simulink model "SymbolSyncTest"  (R2022b)
settings: Solver=VariableStepAuto  StartTime=0.0  StopTime=10.0  RelTol=1e-3
libraries: commfilt2 x2, commrandsrc3 x1, commdigbbndpm3 x1, dspsigops x1
settings Model: Creator=svdvl  LastModifiedBy=User

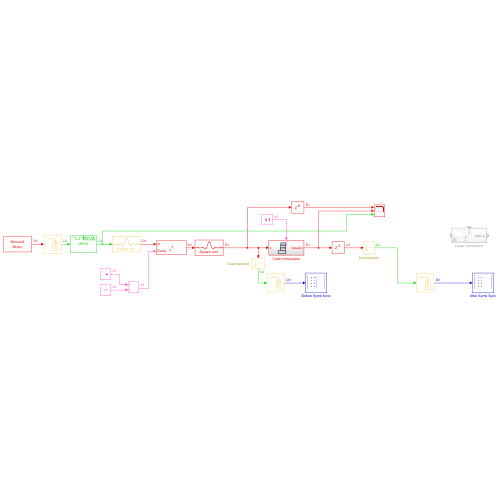
[thumbnail: Simulink's stored preview of the top-level diagram]
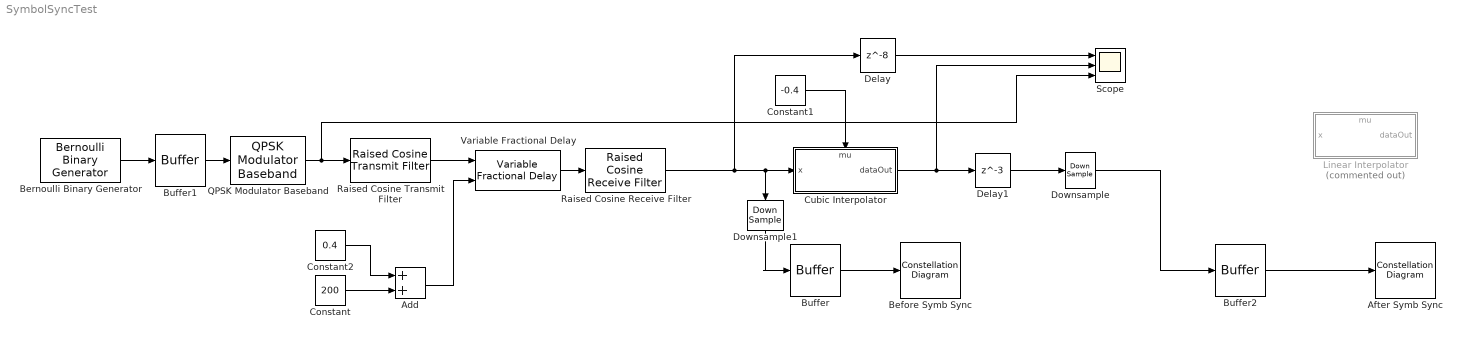
== system SymbolSyncTest ==
  Add : Sum
  After Symb Sync : ConstellationDiagram  WindowPosition=[1026.000000,90.000000,600.000000,600.000000,]  ScopeFrameLocation=window  DefaultConfigurationName=comm.scopes.ConstellationDiagramBlockCfg
  Before Symb Sync : ConstellationDiagram  WindowPosition=[382.000000,84.000000,600.000000,600.000000,]  ScopeFrameLocation=window  DefaultConfigurationName=comm.scopes.ConstellationDiagramBlockCfg
  Bernoulli Binary Generator : commrandsrc3/Bernoulli Binary Generator  ProbabilityOfZero=0.5  SeedSource=Auto  Seed=0  SampleTime=1e-3  SamplesPerFrame=1  OutputDataType=double  SimulateUsing=Interpreted execution
  Buffer : Buffer  N=500  OutputFrames=off
  Buffer1 : Buffer  N=2  OutputFrames=off
  Buffer2 : Buffer  N=500  OutputFrames=off
  Constant : Constant  Value=200
  Constant1 : Constant  Value=-0.4
  Constant2 : Constant  Value=0.4
  Cubic Interpolator : Subsystem
      settings: PortSchema="{\"entries\":[{\"content\":{\"sides\":[{\"content\":{\"connectorIds\":[\"In1\"]},\"type\":\"ConnectorPlacement.EquallySpacedRectSide\",\"uuid\":\"e185856d-5f81-4c71-aeba-8657e8be69b7\"},{\"content\":{\"connectorIds\":[\"Out1\"],\"side\":\"RIGHT\"},\"type\":\"ConnectorPlacement.EquallySpacedRectSide\",\"uuid\":\"487ec109-4505-4025-a071-939a946bead6\"},{\"content\":{\"connectorIds\":[\"In2\"],\"side\":\"TOP\"},\"type\":\"ConnectorPlacement.EquallySpacedRectSide\",\"uuid\":\"bdbbf84f-c060-4097-b440-093ef9dcf44f\"},{\"content\":{\"connectorIds\":[],\"side\":\"BOTTOM\"},\"type\":\"ConnectorPlacement.EquallySpacedRectSide\",\"uuid\":\"14959837-ab14-4ae0-ae0e-9624de46668b\"}]},\"type\":\"ConnectorPlacement.EquallySpacedConnector\",\"uuid\":\"80c256de-e921-4425-90d6-76c464211f17\"}],\"packageUris\":[\"http://schema.mathworks.com/mf0/Connector/R2020b\"],\"version\":\"1.0\"}"
  Delay : Delay  DelayLength=8
  Delay1 : Delay  DelayLength=3
  Downsample : DownSample  RateOptions=Allow multirate processing
  Downsample1 : DownSample  RateOptions=Allow multirate processing
  Linear Interpolator : Subsystem  Commented=on
      settings: PortSchema="{\"entries\":[{\"content\":{\"sides\":[{\"content\":{\"connectorIds\":[\"In1\"]},\"type\":\"ConnectorPlacement.EquallySpacedRectSide\",\"uuid\":\"e185856d-5f81-4c71-aeba-8657e8be69b7\"},{\"content\":{\"connectorIds\":[\"Out1\"],\"side\":\"RIGHT\"},\"type\":\"ConnectorPlacement.EquallySpacedRectSide\",\"uuid\":\"487ec109-4505-4025-a071-939a946bead6\"},{\"content\":{\"connectorIds\":[\"In2\"],\"side\":\"TOP\"},\"type\":\"ConnectorPlacement.EquallySpacedRectSide\",\"uuid\":\"bdbbf84f-c060-4097-b440-093ef9dcf44f\"},{\"content\":{\"connectorIds\":[],\"side\":\"BOTTOM\"},\"type\":\"ConnectorPlacement.EquallySpacedRectSide\",\"uuid\":\"14959837-ab14-4ae0-ae0e-9624de46668b\"}]},\"type\":\"ConnectorPlacement.EquallySpacedConnector\",\"uuid\":\"80c256de-e921-4425-90d6-76c464211f17\"}],\"packageUris\":[\"http://schema.mathworks.com/mf0/Connector/R2020b\"],\"version\":\"1.0\"}"
  QPSK Modulator Baseband : commdigbbndpm3/QPSK Modulator Baseband  InType=Bit  Enc=Gray  Ph=pi/4  outDtype=double  outWordLen=16  outUDDataType=sfix(16)  outFracLenMode=Best precision  outFracLen=15  outDataTypeStr=double  outLastDataTypeStr=double
      settings: LibrarySourceBlock=|
      | commhdldigbbndpm/QPSK
      | Modulator
      | Baseband
  Raised Cosine Receive Filter : commfilt2/Raised Cosine Receive Filter  filtType=Square root  R=0.2  filtSpan=20  N=2  downFactor=1  downOffset=0  filterGain=1  RateOptions=Allow multirate processing  framing=Mute  checkCoeff=off  variableName=rcRxFilt  currentFiltSpan=10  D=5  inputOffset=0  sampMode=Mute  saveAsFlag=0  rateMode=Downsampling  checkGain=Normalized  launchFVT=on  roundingMode=Floor  overflowMode=off  coeffDataTypeStr=Inherit: Same word length as input  coeffMin=[]  coeffMax=[]  coeffLastDataTypeStr=Inherit: Same word length as input  accumDataTypeStr=Inherit: Same as product output  accumLastDataTypeStr=Inherit: Same as product output  outputDataTypeStr=Inherit: Same as accumulator  outputMin=[]  outputMax=[]  outputLastDataTypeStr=Inherit: Same as accumulator
      settings: LibrarySourceBlock=|
      | commhdlfilt/Raised Cosine
      | Receive Filter
  Raised Cosine Transmit Filter : commfilt2/Raised Cosine Transmit Filter  filtType=Square root  R=0.2  filtSpan=20  N=2  filterGain=1  RateOptions=Allow multirate processing  framing=Mute  checkCoeff=off  variableName=rcTxFilt  checkGain=Normalized  sampMode=Mute  saveAsFlag=0  currentFiltSpan=10  D=5  launchFVT=on  roundingMode=Floor  overflowMode=off  coeffDataTypeStr=Inherit: Same word length as input  coeffMin=[]  coeffMax=[]  coeffLastDataTypeStr=Inherit: Same word length as input  outputDataTypeStr=Inherit: Same as accumulator  outputMin=[]  outputMax=[]  outputLastDataTypeStr=Inherit: Same as accumulator
      settings: LibrarySourceBlock=|
      | commhdlfilt/Raised Cosine
      | Transmit Filter
  Scope : Scope  NumInputPorts=3
  Variable Fractional Delay : dspsigops/Variable Fractional Delay  mode=OBSOLETE  modeActive=FIR  L=200  FarrowL=400  R=110  alpha=1  dmax=220  ic=0  noDFT=off  fallbackFIR=Clip to the minimum value necessary for centered kernel  fallbackFarrow=Clip to the minimum value necessary for centered kernel  roundingMode=Zero  overflowMode=off
  wires:
  Bernoulli Binary Generator/1 -> Buffer1/1
  QPSK Modulator Baseband/1 -> Scope/3, Raised Cosine Transmit Filter/1
  Raised Cosine Transmit Filter/1 -> Variable Fractional Delay/1
  Variable Fractional Delay/1 -> Raised Cosine Receive Filter/1
  Buffer/1 -> Before Symb Sync/1
  Buffer1/1 -> QPSK Modulator Baseband/1
  Constant1/1 -> Cubic Interpolator/2(mu)
  Buffer2/1 -> After Symb Sync/1
  Cubic Interpolator/1(dataOut) -> Scope/2, Delay1/1
  Downsample/1 -> Buffer2/1
  Downsample1/1 -> Buffer/1
  Delay/1 -> Scope/1
  Constant/1 -> Add/2
  Constant2/1 -> Add/1
  Add/1 -> Variable Fractional Delay/2
  Raised Cosine Receive Filter/1 -> Cubic Interpolator/1(x), Downsample1/1, Delay/1
  Delay1/1 -> Downsample/1

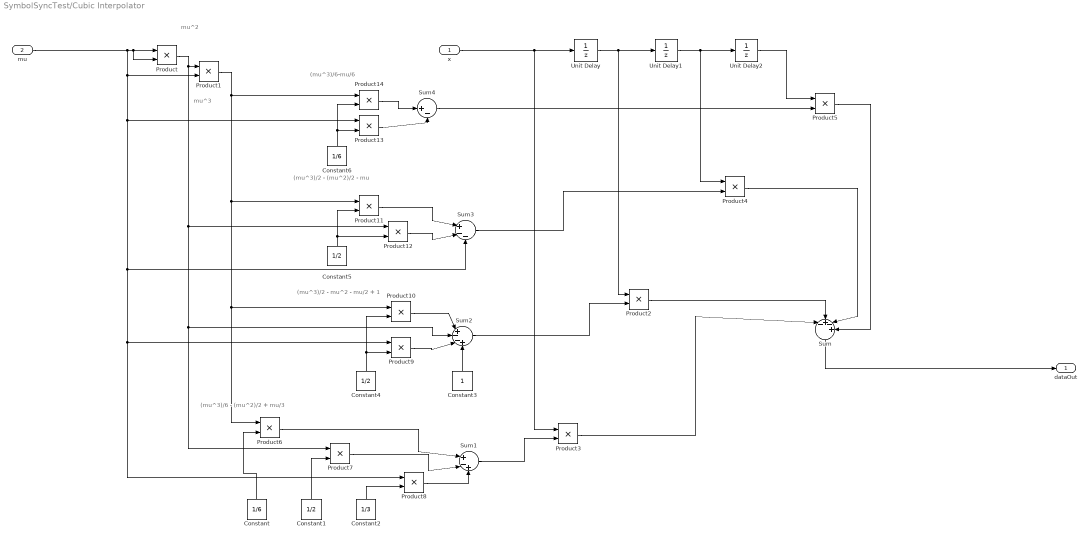
== system SymbolSyncTest/Cubic Interpolator ==
  note: (mu^3)/6-mu/6
  note: (mu^3)/2 - (mu^2)/2 - mu
  note: (mu^3)/2 - mu^2 - mu/2 + 1
  note: (mu^3)/6 - (mu^2)/2 + mu/3
  note: mu^2
  note: mu^3
  x : Inport
  mu : Inport  Port=2
  Constant : Constant  Value=1/6  SampleTime=-1
  Constant1 : Constant  Value=1/2  SampleTime=-1
  Constant2 : Constant  Value=1/3  SampleTime=-1
  Constant3 : Constant  SampleTime=-1
  Constant4 : Constant  Value=1/2  SampleTime=-1
  Constant5 : Constant  Value=1/2  SampleTime=-1
  Constant6 : Constant  Value=1/6  SampleTime=-1
  Product{,1..14} (15 alike) : Product
  Sum : Sum  Inputs=|-+-+
  Sum1 : Sum  Inputs=|+-+
  Sum2 : Sum  Inputs=|+--+
  Sum3 : Sum  Inputs=|+--
  Sum4 : Sum  Inputs=|+-
  Unit Delay : UnitDelay  SampleTime=-1  HasFrameUpgradeWarning=on
  Unit Delay1 : UnitDelay  SampleTime=-1  HasFrameUpgradeWarning=on
  Unit Delay2 : UnitDelay  SampleTime=-1  HasFrameUpgradeWarning=on
  dataOut : Outport
  wires:
  Sum/1 -> dataOut/1
  mu/1 -> Product/2, Product/1, Product13/1, Sum3/3, Product9/1, Product8/1, Product1/2
  Product/1 -> Product12/1, Sum2/2, Product7/1, Product1/1
  Unit Delay/1 -> Product2/1, Unit Delay1/1
  Unit Delay1/1 -> Product4/1, Unit Delay2/1
  Unit Delay2/1 -> Product5/1
  x/1 -> Product3/1, Unit Delay/1
  Product3/1 -> Sum/1
  Product2/1 -> Sum/2
  Product4/1 -> Sum/3
  Product5/1 -> Sum/4
  Constant/1 -> Product6/2
  Product1/1 -> Product11/1, Product10/1, Product6/1, Product14/1
  Constant1/1 -> Product7/2
  Constant2/1 -> Product8/2
  Product7/1 -> Sum1/2
  Sum1/1 -> Product3/2
  Product8/1 -> Sum1/3
  Product6/1 -> Sum1/1
  Constant3/1 -> Sum2/4
  Constant4/1 -> Product10/2, Product9/2
  Product9/1 -> Sum2/3
  Product10/1 -> Sum2/1
  Sum2/1 -> Product2/2
  Constant5/1 -> Product11/2, Product12/2
  Product12/1 -> Sum3/2
  Product11/1 -> Sum3/1
  Sum3/1 -> Product4/2
  Constant6/1 -> Product14/2, Product13/2
  Product14/1 -> Sum4/1
  Product13/1 -> Sum4/2
  Sum4/1 -> Product5/2

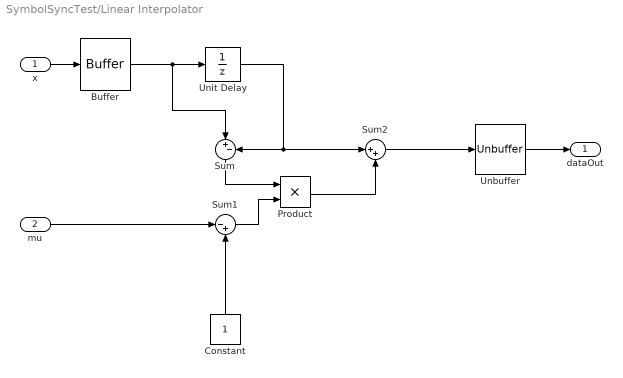
== system SymbolSyncTest/Linear Interpolator ==
  x : Inport
  mu : Inport  Port=2
  Buffer : Buffer  N=4  OutputFrames=off
  Constant : Constant  SampleTime=-1
  Product : Product
  Sum : Sum  Inputs=|+-
  Sum1 : Sum  Inputs=|-+
  Sum2 : Sum  Inputs=|++
  Unbuffer : Unbuffer
  Unit Delay : UnitDelay  SampleTime=-1  HasFrameUpgradeWarning=on
  dataOut : Outport
  wires:
  Unit Delay/1 -> Sum/2, Sum2/1
  Sum1/1 -> Product/2
  Sum/1 -> Product/1
  mu/1 -> Sum1/1
  Sum2/1 -> Unbuffer/1
  x/1 -> Buffer/1
  Constant/1 -> Sum1/2
  Product/1 -> Sum2/2
  Buffer/1 -> Sum/1, Unit Delay/1
  Unbuffer/1 -> dataOut/1
